simulink model "Model"  (R2023b)
settings: Solver=VariableStepAuto  StartTime=0.0  StopTime=1  RelTol=1e-6
values from neighbouring files (symbols this model uses):
  A = inv(K)*A    [SSA.m]
  B_ss = inv(K)*B_ss    [SSA.m]
  C = d.NominalValue*C1 + dp.NominalValue*C2    [SSA.m]
  D_ss = [D,F]    [SSA.m]
  Tsc = 1/5000    (= 0.0002)    [init_controller.m]
undefined symbols (not defined in the file or in its folder): DiscIntNeverNeededParam
libraries: simulink x1
settings Model: Creator=maxim  LastModifiedBy=maxim
settings OptimizationCC: ReuseModelBlockBuffer=off

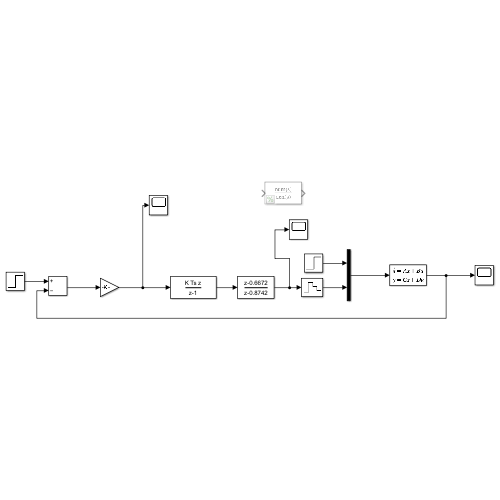
[thumbnail: Simulink's stored preview of the top-level diagram]
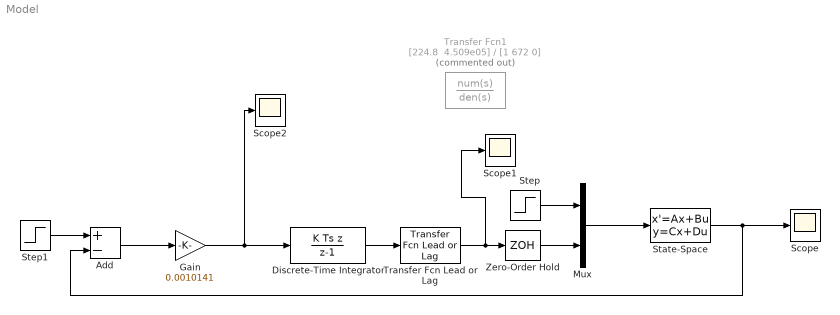
== system Model ==
  Add : Sum  Inputs=+-
  Discrete-Time Integrator : DiscreteIntegrator  IntegratorMethod=Integration: Backward Euler  gainval=1  SampleTime=Tsc  ICPrevOutput=DiscIntNeverNeededParam  ICPrevScaledInput=DiscIntNeverNeededParam
  Gain : Gain  Gain=0.0010141
  Mux : Mux  Inputs=2
  Scope : Scope
  Scope1 : Scope
  Scope2 : Scope
  State-Space : StateSpace  A=A.Nominal  B=B_ss.Nominal  C=C  D=D_ss.Nominal  InitialCondition=0
  Step : Step  Time=0.3  Before=30  After=45  SampleTime=0
  Step1 : Step  Time=0.2  Before=60  After=130  SampleTime=0
  Transfer Fcn Lead or Lag : simulink/Discrete/Transfer Fcn Lead or Lag  PoleZ=0.8742  ZeroZ=0.6672  ICPrevOutput=0.0  ICPrevInput=0.0  DoSatur=off
  Transfer Fcn1 : TransferFcn  Commented=on  Numerator="[224.8  4.509e05]"  Denominator=[1 672 0]
  Zero-Order Hold : ZeroOrderHold  SampleTime=Tsc
  wires:
  Step/1 -> Mux/1
  Mux/1 -> State-Space/1
  State-Space/1 -> Add/2, Scope/1
  Transfer Fcn Lead or Lag/1 -> Scope1/1, Zero-Order Hold/1
  Step1/1 -> Add/1
  Discrete-Time Integrator/1 -> Transfer Fcn Lead or Lag/1
  Add/1 -> Gain/1
  Zero-Order Hold/1 -> Mux/2
  Gain/1 -> Scope2/1, Discrete-Time Integrator/1
